simulink model "external_sim_Planar3DoF"  (R2023a)
settings: Solver=FixedStepAuto  StartTime=0.0  StopTime=5  FixedStep=0.001  RelTol=1e-3
values from neighbouring files (symbols this model uses):
  ROBOT = Planar3DoF(rho, radius, arm_length)    [calcSysMatrices.m]    (also in init_sim_Planar6DoF.m = Planar6DoF(m_fac, m_EE, com_EE, I_EE); robot_chain_dynamics.m = Planar_n_DoF(rho, radius, arm_length, num_links))
libraries: robotmaniplib x1
settings Model: Creator=wu_xw  LastModifiedBy=divij
settings SolverCC: AlgebraicLoopSolver=TrustRegion
settings DataIOCC: ReturnWorkspaceOutputs=off
settings DebuggingCC: UnconnectedInputMsg=warning  UnconnectedOutputMsg=warning  UnconnectedLineMsg=warning  ArithmeticOperatorsInVariantConditions=warning
settings ModelReferenceCC: EnableRefExpFcnMdlSchedulingChecks=on
settings SFSimCC: SimUseLocalCustomCode=off  CustomCodeUndefinedFunction=UseInterfaceOnly
settings RTWCC: RTWUseLocalCustomCode=off

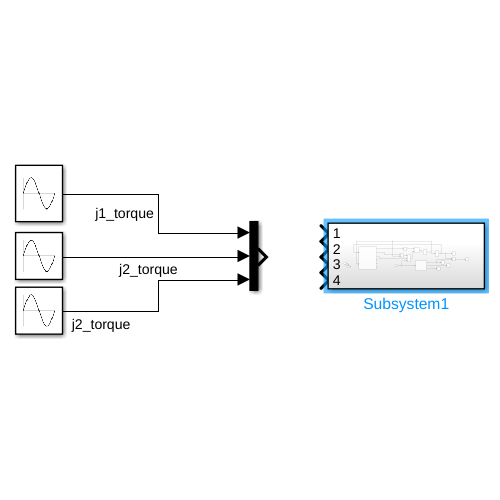
[thumbnail: Simulink's stored preview of the top-level diagram]
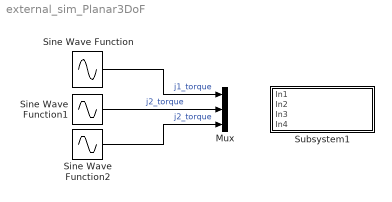
== system external_sim_Planar3DoF ==
  Mux : Mux  Inputs=3
  Sine Wave Function : Sin  Amplitude=2  SampleTime=0
  Sine Wave Function1 : Sin  SampleTime=0
  Sine Wave Function2 : Sin  Amplitude=0.5  SampleTime=0
  Subsystem1 : Subsystem
  wires:
  Sine Wave Function1/1 -> Mux/2  "j2_torque"
  Sine Wave Function2/1 -> Mux/3  "j2_torque"
  Sine Wave Function/1 -> Mux/1  "j1_torque"

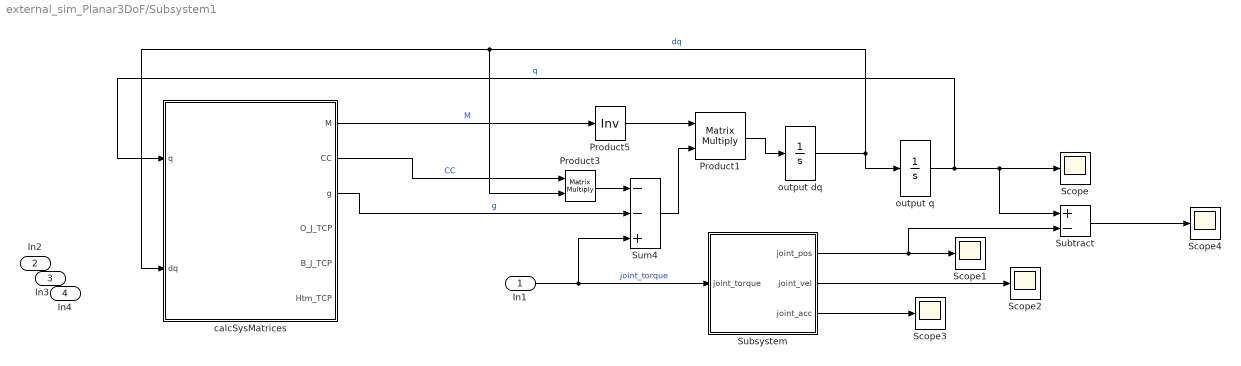
== system external_sim_Planar3DoF/Subsystem1 ==
  In1 : Inport
  In2 : Inport  Port=2
  In3 : Inport  Port=3
  In4 : Inport  Port=4
  Product1 : Product  Multiplication=Matrix(*)  RndMeth=Zero
  Product3 : Product  Multiplication=Matrix(*)  RndMeth=Zero
  Product5 : Product  Inputs=/  Multiplication=Matrix(*)  RndMeth=Zero
  Scope{,1..4} (5 alike) : Scope
  Subsystem : Subsystem
  Subtract : Sum  Inputs=+-
  Sum4 : Sum  Inputs=--+
  calcSysMatrices : MATLAB Function  TreatAsAtomicUnit=on  mask{ROBOT=ROBOT}
      mask prompts: ROBOT "Robot Model"
      mask help:
      | Calculates inertia and coriolis compensation matrices
      |
      | A MATLAB structure ROBOT with the fields:
      |
      | g0 - matrix stacking vertically the homogeneous transformation matrices from parent to link in the zero-configuration
      | csi - vector stacking vertically the 6-by-1 relative body jacobian (twist) in link frame
      | Mass - block diagonal matrix, where each block is the 6-by-6 inertia matrix of the link in link frame
      |
      | must be initialized in workspace.
  output dq : Integrator  UpperSaturationLimit=10  LowerSaturationLimit=-10
  output q : Integrator  LimitOutput=on  UpperSaturationLimit=pi/2  LowerSaturationLimit=-pi/2
  wires:
  Sum4/1 -> Product1/2
  Product5/1 -> Product1/1
  output q/1 -> calcSysMatrices/1(q), Subtract/1, Scope/1  "q"
  Product3/1 -> Sum4/1
  calcSysMatrices/2(CC) -> Product3/1  "CC"
  calcSysMatrices/1(M) -> Product5/1  "M"
  output dq/1 -> calcSysMatrices/2(dq), Product3/2, output q/1  "dq"
  Product1/1 -> output dq/1
  calcSysMatrices/3(g) -> Sum4/2  "g"
  Subsystem/1(joint_pos) -> Subtract/2, Scope1/1
  Subsystem/3(joint_acc) -> Scope3/1
  Subsystem/2(joint_vel) -> Scope2/1
  In1/1 -> Subsystem/1(joint_torque), Sum4/3  "joint_torque"
  Subtract/1 -> Scope4/1

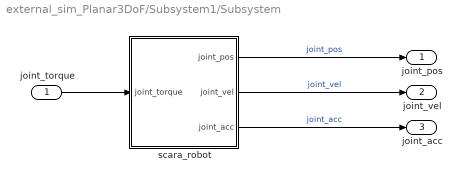
== system external_sim_Planar3DoF/Subsystem1/Subsystem ==
  joint_torque : Inport
  scara_robot : Subsystem  TreatAsAtomicUnit=on
  joint_pos : Outport
  joint_vel : Outport  Port=2
  joint_acc : Outport  Port=3
  wires:
  scara_robot/3(joint_acc) -> joint_acc/1  "joint_acc"
  scara_robot/2(joint_vel) -> joint_vel/1  "joint_vel"
  scara_robot/1(joint_pos) -> joint_pos/1  "joint_pos"
  joint_torque/1 -> scara_robot/1(joint_torque)

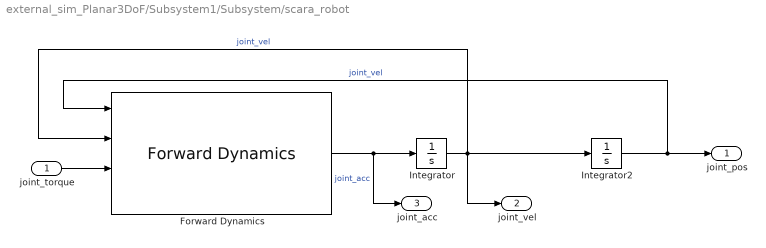
== system external_sim_Planar3DoF/Subsystem1/Subsystem/scara_robot ==
  joint_torque : Inport
  Forward Dynamics : robotmaniplib/Forward Dynamics  RigidBodyTree=robot  SimulateUsing=Interpreted execution
  Integrator : Integrator  UpperSaturationLimit=10  LowerSaturationLimit=-10
  Integrator2 : Integrator  LimitOutput=on  UpperSaturationLimit=pi/2  LowerSaturationLimit=-pi/2
  joint_pos : Outport
  joint_vel : Outport  Port=2
  joint_acc : Outport  Port=3
  wires:
  Forward Dynamics/1 -> joint_acc/1, Integrator/1  "joint_acc"
  Integrator/1 -> Integrator2/1, joint_vel/1, Forward Dynamics/2  "joint_vel"
  joint_torque/1 -> Forward Dynamics/3
  Integrator2/1 -> Forward Dynamics/1, joint_pos/1  "joint_vel"

== matlab function external_sim_Planar3DoF/Subsystem1/calcSysMatrices ==
  data: q input; M output size=3,3; dq input; CC output; ROBOT parameter; g output; O_J_TCP output; B_J_TCP output; Htm_TCP output
%%%%%%%%%%%%%%%%%%%%%%%%%%%%%%%%%%%%%%%%%%
% Calculation of system matrices
%%%%%%%%%%%%%%%%%%%%%%%%%%%%%%%%%%%%%%%%%%
%
% Calculates the dynamic and kinematic matrices by using the iterative 
% algorithm proposed in [1]. Kinematic and inertia parameters of the robot 
% can be given in a compact way. Additionally, this algorithm can ensure 
% the skew-symmetric property of dM - 2C.
%
% Inputs:
% q:        Current joint positions, n-by-1 vector
% dq:       Current joint velocities, n-by-1 vector
% ROBOT:    Robot parameters, MATLAB structure with three
%           fields:
%           g0:       4n-by-4 matrix stacking vertically the homogeneous
%                     transformation matrices from parent to link in the
%                     zero-configuration
%           csi:      6n-by-1 vector stacking vertically the 6-by-1 
%                     relative body jacobian (twist)
%           Mass:     6n-by-6 matrix stacking vertically the 6-by-6   
%                     constant body inertia matrix from parent to link
%           g_vec:    3-by-1 gravitational acceleration constant
%           tcp_t_ee: 4-by-4 homogeneous transformation matrix from 
%                     end-effector to tcp
%
% Outputs
% M:        n-by-n joint space inertia matrix
% CC:       n-by-n joint space Cor./centrifugal matrix
% g:        n-by-1 gravity torque vector
% O_J_TCP:  6-by-n hybrid jacobian of tcp
% B_J_TCP:  6-by-n body jacobian of tcp
% Htm_TCP:  4-by-4 homogeneous transformation matrix from tcp to base
%
% References
% [1] Garofalo, Gianluca, Christian Ott and Alin Albu-Schäffer. "On the
% closed form computation of the dynamic matrices and their differentiations."
% 2013 IEEE/RSJ International Conference on Intelligent Robots and Systems
% (2013): 2364-2359.
%
% Implemented by Xuwei Wu.

function [M, CC, g, O_J_TCP, B_J_TCP, Htm_TCP] = calcSysMatrices(q, dq, ROBOT)
%#codegen

% reshape signals
ndof = size(ROBOT.g0, 1)/4;
q = reshape(q, ndof, 1);
dq = reshape(dq, ndof, 1);

% pre-allocate memory for variables
M = zeros(ndof, ndof);
dM = zeros(ndof, ndof);
CC = zeros(ndof, ndof);
g = zeros(ndof, 1);
J_pre = zeros(6, ndof);
dJ_pre = zeros(6, ndof);
inertialTwist_pre = zeros(6,1);
O_Htm_pre = eye(4);

% iterate from the root to the end-effector of the serial manipulator
for iLink = 1:ndof
    
    % initialize indices of the current iteration
    idxStart_4Row = 4*(iLink-1) + 1;
    idxEnd_4Row = idxStart_4Row + 3;
    idxStart_6Row = 6*(iLink-1) + 1;
    idxEnd_6Row = idxStart_6Row + 5;
    
    % compute relative body twist
    relBodyJac = ROBOT.csi(idxStart_6Row:idxEnd_6Row);
    relBodyJac = reshape(relBodyJac, 6, 1);
    relTwist = relBodyJac * dq(iLink);
    
    % compute relative homogeneous transformation matrix between link and
    % its parent
    Htm = ROBOT.g0(idxStart_4Row:idxEnd_4Row, 1:4);
    Htm = Htm * Exponential(relBodyJac, q(iLink));
    
    % propagate rotation matrix, body twists, body jacobians and 
    % derivatives of body jacobians
    O_Htm = O_Htm_pre * Htm;
    inertialTwist = relTwist;
    invAd = InvAdjoint(Htm);
    J = zeros(6, ndof);
    dJ = zeros(6, ndof);
    if iLink > 1
        inertialTwist = inertialTwist + invAd * inertialTwist_pre;
        J(1:6, 1:iLink-1) = invAd * J_pre(1:6, 1:iLink-1);
        dJ(1:6, 1:iLink-1) = invAd * dJ_pre(1:6, 1:iLink-1)- LieBracket(relTwist) * J(1:6, 1:iLink-1);
    end
    J(1:6, iLink) = relBodyJac;
    
    % update inertia matrix
    tmp = J(1:6, 1:iLink)' * ROBOT.Mass(idxStart_6Row:idxEnd_6Row, 1:6);
    M(1:iLink, 1:iLink) = M(1:iLink, 1:iLink) + tmp * J(1:6, 1:iLink);
    tmptmp = tmp * dJ(1:6, 1:iLink);
    dM(1:iLink, 1:iLink) = dM(1:iLink, 1:iLink) + tmptmp + tmptmp';
    
    % update Cor.\centrifugal matrix
    % Method 1: Original version from [1]
    % Mass_x_ad_tmp = ROBOT.Mass(idxStart_6Row:idxEnd_6Row, 1:6) * LieBracket(inertialTwist);
    % Mass_x_ad_tmp = Mass_x_ad_tmp - Mass_x_ad_tmp';
    Mass_x_ad_tmp = SkewCoriolis(ROBOT.Mass(idxStart_6Row:idxEnd_6Row, 1:6), inertialTwist(4:6));
    CC(1:iLink, 1:iLink) = CC(1:iLink, 1:iLink) + J(1:6, 1:iLink)' * Mass_x_ad_tmp * J(1:6, 1:iLink) + tmp * dJ(1:6, 1:iLink);
    
    % update gravity torque vector
    g(1:iLink) = g(1:iLink) + tmp(1:iLink, 1:3) * O_Htm(1:3, 1:3)' * ROBOT.g_vec;
    
    % update variables of parent link
    J_pre = J;
    dJ_pre = dJ;
    inertialTwist_pre = inertialTwist;
    O_Htm_pre = O_Htm;
end
Htm_TCP = O_Htm(1:4,1:4) * ROBOT.tcp_t_ee;
B_J_TCP = InvAdjoint(ROBOT.tcp_t_ee) * J(1:6, 1:ndof);
O_J_TCP = [Htm_TCP(1:3, 1:3)* B_J_TCP(1:3, 1:ndof);Htm_TCP(1:3, 1:3)*B_J_TCP(4:6, 1:ndof)];
end

function out = Skew(vec)
% Skew operator
% Implemented by Gianluca Garofalo.

out = [
    0         -vec(3)   vec(2)
    vec(3)    0         -vec(1)
    -vec(2)   vec(1)    0
    ];

end

function out = SkewCoriolis(Mass, w)
Sw = Skew(w);
tmp = Mass(4:6, 1:3)*Sw;
tmp2 = Mass(4:6, 4:6)*Sw;
out = [Mass(1,1)*Sw -tmp'; tmp tmp2 - tmp2'];
end

function out = Exponential(csi, theta)
% Twist exponential of the relative body jacobian
% Implemented by Gianluca Garofalo.

o = [0 0 0].';
I = eye( 3 );
v = csi(1:3);
w = csi(4:6);
if all( w == o )
    out = [I v*theta; zeros(1,3) 1];
else
    w_hat = Skew( w );
    R_minus_I = w_hat * sin( theta ) + w_hat * w_hat * ( 1 - cos(theta) );
    out = [I+R_minus_I zeros(3,1); zeros(1,3) 1];
end
end

function out = InvAdjoint(Htm)
% Inverse of the adjoint transformation
% Implemented by Gianluca Garofalo.

R_tra = Htm(1:3,1:3).';
p_hat = Skew( Htm(1:3,4) );
out = [R_tra -R_tra*p_hat; zeros(3) R_tra];
end

function ad = LieBracket(twist)
% Lie bracket of the body twist
% Implemented by Gianluca Garofalo.

Sv = Skew( twist(1:3) );
Sw = Skew( twist(4:6) );
ad = [Sw Sv; zeros(3) Sw];
end
